simulink library "vhcl1turb_cl"  (R2022a)
settings: Solver=VariableStepAuto  StartTime=0.0  StopTime=10.0  RelTol=1e-3
undefined symbols (not defined in the file): env, VEHICLE, vhcl
libraries: vrlib x2, addedMass_cl x1, dragTurbineManta_ul x1, fluidDynamicSurface_cl x1, fuselage_cl x1, sixDoFDynamics_cl x1, tethersMoment_cl x1, thrAttachPtKinematics_ul x1
settings Model: Creator=mcobb  LastModifiedBy=lhill8
settings SolverCC: AlgebraicLoopSolver=TrustRegion
settings DebuggingCC: UnconnectedInputMsg=warning  UnconnectedOutputMsg=warning  UnconnectedLineMsg=warning  SFMachineParentedDataDiag=warning  ArithmeticOperatorsInVariantConditions=warning
settings SFSimCC: CustomCodeUndefinedFunction=UseInterfaceOnly

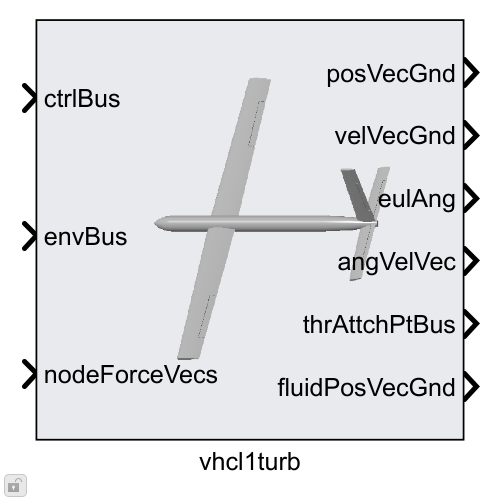
[thumbnail: Simulink's stored preview of the top-level diagram]
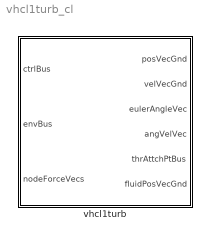
== system vhcl1turb_cl ==
  vhcl1turb : Subsystem  VariantControl=strcmpi(VEHICLE,'vehicleManta')  mask{vcl=vhcl, rho=env.water.density.Value, grav=env.gravAccel.Value}
      mask prompts: vcl "Vehicle"; rho "Density"; grav "Gravity"
      mask DialogControl Container9 Prompt: General
      mask DialogControl Container5 Prompt: Vehicle object (OCT.vehicle)
      mask DialogControl ParameterGroupVar Prompt: Environment Object (OCT.env)
      mask Display:
      | image('kite2.PNG',[0 0 700 700]/4,'on')
      | 
      | port_label('input',1,'ctrlBus')
      | port_label('input',2,'envBus')
      | port_label('input',3,'nodeForceVecs')
      | 
      | port_label('output',1,'posVecGnd')
      | port_label('output',2,'velVecGnd')
      | port_label('output',3,'eulAng')
      | port_label('output',4,'angVelVec')
      | port_label('output',5,'thrAttchPtBus')
      | port_label('output',6,'fluidPosVecGnd')

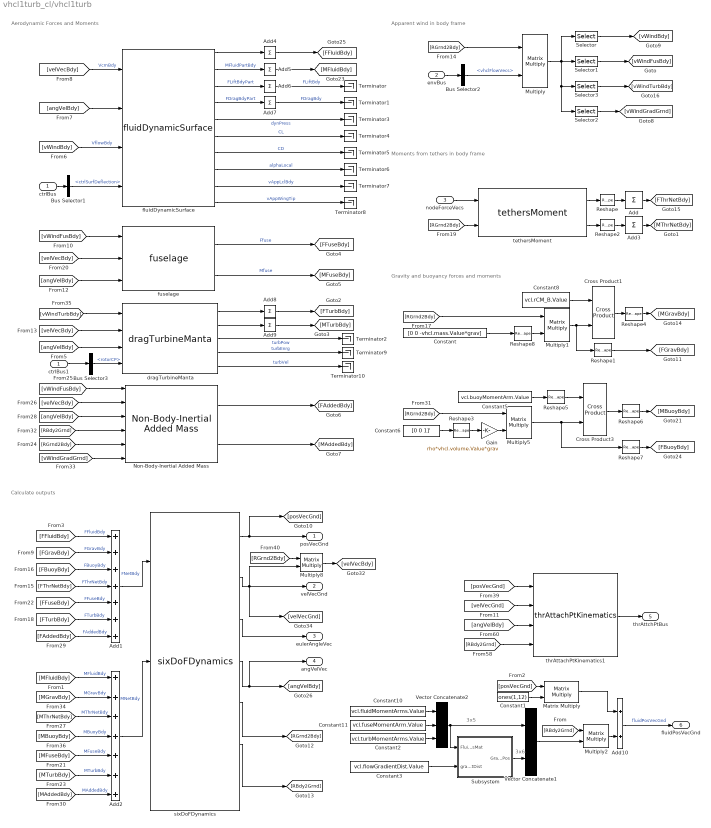
== system vhcl1turb_cl/vhcl1turb ==
  note: Aerodynamic Forces and Moments
  note: Moments from tethers in body frame
  note: Gravity and buoyancy forces and moments
  note: Apparent wind in body frame
  note: Calculate outputs
  note: 3x5
  note: 3x6
  ctrlBus : Inport  OutDataTypeStr=Bus: fltCtrlBus
  envBus : Inport  Port=2  OutDataTypeStr=Bus: envBus
  nodeForceVecs : Inport  Port=3
  Add : Sum  Inputs=+  CollapseMode=Specified dimension  CollapseDim=2
  Add1 : Sum  Inputs=+++++++
  Add10 : Sum
  Add2 : Sum  Inputs=+++++++
  Add3 : Sum  Inputs=+  CollapseMode=Specified dimension  CollapseDim=2
  Add{4..9} (6 alike) : Sum  Inputs=1  CollapseMode=Specified dimension  CollapseDim=2
  Bus Selector1 : BusSelector  OutputSignals=ctrlSurfDeflection
  Bus Selector2 : BusSelector  OutputSignals=vhclFlowVecs
  Bus Selector3 : BusSelector  OutputSignals=rotorCP
  Constant : Constant  Value=[0 0 -vhcl.mass.Value*grav]
  Constant1 : Constant  Value=ones(1,12)  VectorParams1D=off
  Constant10 : Constant  Value=vcl.fluidMomentArms.Value
  Constant11 : Constant  Value=vcl.fuseMomentArm.Value
  Constant2 : Constant  Value=vcl.turbMomentArms.Value
  Constant3 : Constant  Value=vcl.flowGradientDist.Value
  Constant5 : Constant  Value=vcl.buoyMomentArm.Value
  Constant6 : Constant  Value=[0 0 1]'
  Constant8 : Constant  Value=vcl.rCM_B.Value
  Cross Product1 : vrlib/Utilities/Cross Product
  Cross Product3 : vrlib/Utilities/Cross Product
  Gain : Gain  Gain=rho*vhcl.volume.Value*grav
  Matrix Multiply : Product  Multiplication=Matrix(*)
  Multiply{,1..2,5,8} (5 alike) : Product  Multiplication=Matrix(*)
  Non-Body-Inertial Added Mass : addedMass_cl/Non-Body-Inertial Added Mass  MaMat=vcl.Ma6x6_LE.Value  rB_LE=vcl.rB_LE.Value  gradDist=vcl.flowGradientDist.Value
  Reshape : Reshape  OutputDimensionality=Customize  OutputDimensions=[3 vcl.numTethers.Value]
  Reshape{1,3..8} (7 alike) : Reshape  OutputDimensionality=Column vector (2-D)
  Reshape2 : Reshape  OutputDimensionality=Customize  OutputDimensions=[3 vcl.numTethers.Value]
  Selector : Selector  NumberOfDimensions=2  InputPortWidth=3  IndexOptions=Select all,Index vector (dialog)  Indices=[1 3],1:4  OutputSizes=1,1
  Selector1 : Selector  NumberOfDimensions=2  InputPortWidth=3  IndexOptions=Select all,Index vector (dialog)  Indices=[1 3],5  OutputSizes=1,1
  Selector2 : Selector  NumberOfDimensions=2  InputPortWidth=3  IndexOptions=Select all,Index vector (dialog)  Indices=[1 3],7:12  OutputSizes=1,1
  Selector3 : Selector  NumberOfDimensions=2  InputPortWidth=3  IndexOptions=Select all,Index vector (dialog)  Indices=[1 3],6  OutputSizes=1,1
  Subsystem : Subsystem
  Terminator{,1..10} (11 alike) : Terminator
  Vector Concatenate1 : Concatenate  Mode=Multidimensional array  ConcatenateDimension=2
  Vector Concatenate2 : Concatenate  NumInputs=3  Mode=Multidimensional array  ConcatenateDimension=2
  ctrlBus1 : InportShadow  OutDataTypeStr=Bus: fltCtrlBus
  dragTurbineManta : dragTurbineManta_ul/dragTurbineManta  rho_fluid=rho  turb_struct=vcl.struct('OCT.turb')
  fluidDynamicSurface : fluidDynamicSurface_cl/fluidDynamicSurface  aeroStruct=vcl.struct('OCT.aeroSurf')  fluidDensity=env.water.density.Value  fluidMomentArms=vcl.fluidMomentArms.Value  fluidRefArea=vcl.fluidRefArea.Value  wingTips=vcl.wingTipPositions.Value
  fuselage : fuselage_cl/fuselage  momArm=vcl.fuseMomentArm.Value  fus=vcl.fuse  fusRhoDa=rho
  sixDoFDynamics : sixDoFDynamics_cl/sixDoFDynamics  vcl=vcl
  tethersMoment : tethersMoment_cl/tethersMoment  arms=vcl.struct('OCT.thrAttch')
  thrAttachPtKinematics1 : thrAttachPtKinematics_ul/thrAttachPtKinematics  atchPts=vcl.struct('OCT.thrAttch')
  posVecGnd : Outport  VectorParamsAs1DForOutWhenUnconnected=off
  velVecGnd : Outport  Port=2  VectorParamsAs1DForOutWhenUnconnected=off
  eulerAngleVec : Outport  Port=3  VectorParamsAs1DForOutWhenUnconnected=off
  angVelVec : Outport  Port=4  VectorParamsAs1DForOutWhenUnconnected=off
  thrAttchPtBus : Outport  Port=5  VectorParamsAs1DForOutWhenUnconnected=off
  fluidPosVecGnd : Outport  Port=6  VectorParamsAs1DForOutWhenUnconnected=off
  wires:
  dragTurbineManta/5 -> Terminator10/1  "turbVel"
  Selector3/1 -> [vWindTurbBdy]
  Constant2/1 -> Vector Concatenate2/3
  ctrlBus1/1 -> Bus Selector3/1
  Bus Selector3/1 -> dragTurbineManta/4  "<rotorCP>"
  dragTurbineManta/4 -> Terminator9/1  "turbEnrg"
  fluidDynamicSurface/10 -> Terminator8/1  "vAppWingTip"
  [posVecGnd] -> Matrix Multiply/1
  Constant1/1 -> Matrix Multiply/2
  Add10/1 -> fluidPosVecGnd/1  "fluidPosVecGnd"
  Matrix Multiply/1 -> Add10/1
  Multiply2/1 -> Add10/2
  [RBdy2Grnd] -> Multiply2/1
  Vector Concatenate1/1 -> Multiply2/2
  Non-Body-Inertial Added Mass/2 -> [MAddedBdy]
  sixDoFDynamics/4 -> angVelVec/1, [angVelBdy]
  Subsystem/1(GradientFlowPos) -> Vector Concatenate1/2
  Constant3/1 -> Subsystem/2(gradientDist)
  Vector Concatenate2/1 -> Subsystem/1(FluidCentPosMat), Vector Concatenate1/1
  Constant11/1 -> Vector Concatenate2/2
  Constant10/1 -> Vector Concatenate2/1
  [RBdy2Grnd] -> thrAttachPtKinematics1/4
  [angVelBdy] -> thrAttachPtKinematics1/3
  [velVecGnd] -> thrAttachPtKinematics1/2
  [posVecGnd] -> thrAttachPtKinematics1/1
  sixDoFDynamics/6 -> [RBdy2Grnd]
  sixDoFDynamics/5 -> [RGrnd2Bdy]
  Add2/1 -> sixDoFDynamics/2  "MNetBdy"
  [MAddedBdy] -> Add2/7  "MAddedBdy"
  [MTurbBdy] -> Add2/6  "MTurbBdy"
  [MFuseBdy] -> Add2/5  "MFuseBdy"
  [MBuoyBdy] -> Add2/4  "MBuoyBdy"
  [MThrNetBdy] -> Add2/3  "MThrNetBdy"
  [MGravBdy] -> Add2/2  "MGravBdy"
  [MFluidBdy] -> Add2/1  "MFluidBdy"
  Add1/1 -> sixDoFDynamics/1  "FNetBdy"
  [FAddedBdy] -> Add1/7  "FAddedBdy"
  [FTurbBdy] -> Add1/6  "FTurbBdy"
  [FFuseBdy] -> Add1/5  "FFuseBdy"
  [FThrNetBdy] -> Add1/4  "FThrNetBdy"
  [FBuoyBdy] -> Add1/3  "FBuoyBdy"
  [FGravBdy] -> Add1/2  "FGravBdy"
  [FFluidBdy] -> Add1/1  "FFluidBdy"
  Multiply8/1 -> [velVecBdy]
  [RGrnd2Bdy] -> Multiply8/1
  Selector2/1 -> [vWindGradGrnd]
  Selector1/1 -> [vWindFusBdy]
  Selector/1 -> [vWindBdy]
  Multiply/1 -> Selector1/1, Selector3/1, Selector2/1, Selector/1
  Bus Selector2/1 -> Multiply/2  "<vhclFlowVecs>"
  envBus/1 -> Bus Selector2/1
  [RGrnd2Bdy] -> Multiply/1
  Add3/1 -> [MThrNetBdy]
  Add/1 -> [FThrNetBdy]
  Reshape2/1 -> Add3/1
  Reshape/1 -> Add/1
  tethersMoment/2 -> Reshape2/1
  tethersMoment/1 -> Reshape/1
  nodeForceVecs/1 -> tethersMoment/1
  [RGrnd2Bdy] -> tethersMoment/2
  Reshape4/1 -> [MGravBdy]
  Cross Product1/1 -> Reshape4/1
  Constant8/1 -> Cross Product1/1
  Reshape8/1 -> Multiply1/2
  [RGrnd2Bdy] -> Multiply1/1
  Constant/1 -> Reshape8/1
  fuselage/2 -> [MFuseBdy]  "Mfuse"
  fuselage/1 -> [FFuseBdy]  "Ffuse"
  Multiply1/1 -> Cross Product1/2, Reshape1/1
  Reshape1/1 -> [FGravBdy]
  Reshape7/1 -> [FBuoyBdy]
  Multiply5/1 -> Cross Product3/2, Reshape7/1
  Reshape6/1 -> [MBuoyBdy]
  Cross Product3/1 -> Reshape6/1
  Reshape5/1 -> Cross Product3/1
  Constant5/1 -> Reshape5/1
  Gain/1 -> Multiply5/2
  [RGrnd2Bdy] -> Multiply5/1
  Reshape3/1 -> Gain/1
  Constant6/1 -> Reshape3/1
  Non-Body-Inertial Added Mass/1 -> [FAddedBdy]
  [vWindGradGrnd] -> Non-Body-Inertial Added Mass/6
  [RGrnd2Bdy] -> Non-Body-Inertial Added Mass/5
  [RBdy2Grnd] -> Non-Body-Inertial Added Mass/4
  [angVelBdy] -> Non-Body-Inertial Added Mass/3
  [velVecBdy] -> Non-Body-Inertial Added Mass/2
  [vWindFusBdy] -> Non-Body-Inertial Added Mass/1
  dragTurbineManta/3 -> Terminator2/1  "turbPow"
  Add9/1 -> [MTurbBdy]
  Add8/1 -> [FTurbBdy]
  dragTurbineManta/2 -> Add9/1
  dragTurbineManta/1 -> Add8/1
  [angVelBdy] -> dragTurbineManta/3
  [velVecBdy] -> dragTurbineManta/2
  [vWindTurbBdy] -> dragTurbineManta/1
  [angVelBdy] -> fuselage/3
  [velVecBdy] -> fuselage/2
  [vWindFusBdy] -> fuselage/1
  ctrlBus/1 -> Bus Selector1/1
  Bus Selector1/1 -> fluidDynamicSurface/4  "<ctrlSurfDeflection>"
  [vWindBdy] -> fluidDynamicSurface/3  "VflowBdy"
  [angVelBdy] -> fluidDynamicSurface/2
  [velVecBdy] -> fluidDynamicSurface/1  "VcmBdy"
  Add7/1 -> Terminator1/1  "FDragBdy"
  Add6/1 -> Terminator/1  "FLiftBdy"
  Add5/1 -> [MFluidBdy]
  Add4/1 -> [FFluidBdy]
  fluidDynamicSurface/9 -> Terminator7/1  "vAppLclBdy"
  fluidDynamicSurface/8 -> Terminator6/1  "alphaLocal"
  fluidDynamicSurface/7 -> Terminator5/1  "CD"
  fluidDynamicSurface/6 -> Terminator4/1  "CL"
  fluidDynamicSurface/5 -> Terminator3/1  "dynPress"
  fluidDynamicSurface/4 -> Add7/1  "FDragBdyPart"
  fluidDynamicSurface/3 -> Add6/1  "FLiftBdyPart"
  fluidDynamicSurface/2 -> Add5/1  "MFluidPartBdy"
  fluidDynamicSurface/1 -> Add4/1
  thrAttachPtKinematics1/1 -> thrAttchPtBus/1
  sixDoFDynamics/2 -> velVecGnd/1, [velVecGnd], Multiply8/2
  sixDoFDynamics/1 -> posVecGnd/1, [posVecGnd]
  sixDoFDynamics/3 -> eulerAngleVec/1

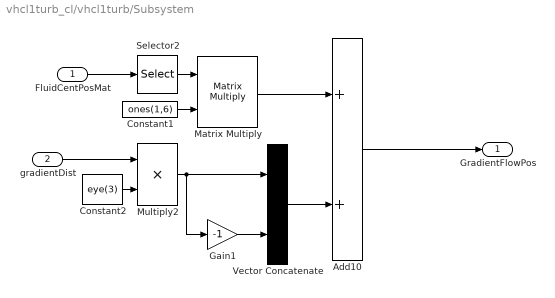
== system vhcl1turb_cl/vhcl1turb/Subsystem ==
  FluidCentPosMat : Inport
  gradientDist : Inport  Port=2
  Add10 : Sum
  Constant1 : Constant  Value=ones(1,6)  VectorParams1D=off
  Constant2 : Constant  Value=eye(3)
  Gain1 : Gain  Gain=-1
  Matrix Multiply : Product  Multiplication=Matrix(*)
  Multiply2 : Product
  Selector2 : Selector  NumberOfDimensions=2  InputPortWidth=3  IndexOptions=Select all,Index vector (dialog)  Indices=[1 3],5  OutputSizes=1,1
  Vector Concatenate : Concatenate  Mode=Multidimensional array  ConcatenateDimension=2
  GradientFlowPos : Outport  VectorParamsAs1DForOutWhenUnconnected=off
  wires:
  gradientDist/1 -> Multiply2/1
  Add10/1 -> GradientFlowPos/1
  Constant2/1 -> Multiply2/2
  Gain1/1 -> Vector Concatenate/2
  Matrix Multiply/1 -> Add10/1
  Constant1/1 -> Matrix Multiply/2
  Multiply2/1 -> Vector Concatenate/1, Gain1/1
  Selector2/1 -> Matrix Multiply/1
  Vector Concatenate/1 -> Add10/2
  FluidCentPosMat/1 -> Selector2/1
